simulink model "model_car"  (R2020a)
settings: Solver=VariableStepAuto  StartTime=0.0  StopTime=100  RelTol=1e-3
libraries: simulink x2
settings Model: Creator=10853  LastModifiedBy=11196

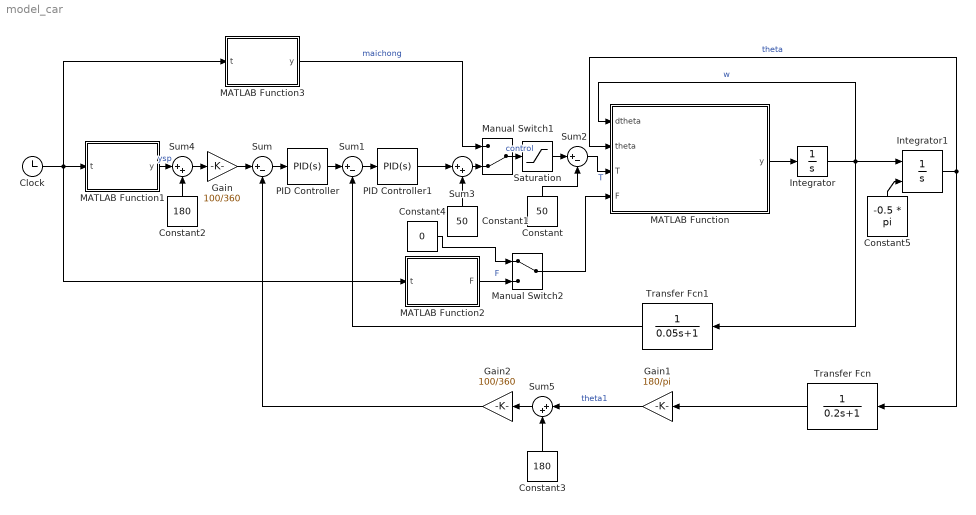
== system model_car ==
  Clock : Clock
  Constant : Constant  Value=50
  Constant1 : Constant  Value=50
  Constant2 : Constant  Value=180
  Constant3 : Constant  Value=180
  Constant4 : Constant  Value=0
  Constant5 : Constant  Value=-0.5 * pi
  Gain : Gain  Gain=100/360
  Gain1 : Gain  Gain=180/pi
  Gain2 : Gain  Gain=100/360
  Integrator : Integrator
  Integrator1 : Integrator  InitialConditionSource=external  InitialCondition=-0.5 * pi  LimitOutput=on  UpperSaturationLimit=pi  LowerSaturationLimit=-pi
  MATLAB Function : MATLAB Function  TreatAsAtomicUnit=on
  MATLAB Function1 : MATLAB Function  TreatAsAtomicUnit=on
  MATLAB Function2 : MATLAB Function  TreatAsAtomicUnit=on
  MATLAB Function3 : MATLAB Function  TreatAsAtomicUnit=on
  Manual Switch1 : ManualSwitch  CurrentSetting=0
  Manual Switch2 : ManualSwitch
  PID Controller : simulink/Continuous/PID Controller  Controller=PID  Form=Parallel  TimeDomain=Continuous-time  UseExternalTs=off  SampleTime=-1  IntegratorMethod=Forward Euler  FilterMethod=Forward Euler  ControllerParametersSource=internal  P=0.8  I=1  D=0.07  UseFilter=on  N=100  TunerSelectOption=Transfer Function Based (PID Tuner App)  InitialConditionSource=internal  InitialConditionForIntegrator=0  InitialConditionForFilter=0  DifferentiatorICPrevScaledInput=0  ExternalReset=none  TrackingMode=off  Kt=1  LimitOutput=off  UpperSaturationLimit=inf  LowerSaturationLimit=-inf  LinearizeAsGain=on  AntiWindupMode=none  Kb=1  POutMin=[]  POutMax=[]  IOutMin=[]  IOutMax=[]  DOutMin=[]  DOutMax=[]  NOutMin=[]  NOutMax=[]  SumOutMin=[]  SumOutMax=[]  SaturationOutMin=[]  SaturationOutMax=[]  PParamMin=[]  PParamMax=[]  IParamMin=[]  IParamMax=[]  DParamMin=[]  DParamMax=[]  NParamMin=[]  NParamMax=[]  KbParamMin=[]  KbParamMax=[]  KtParamMin=[]  KtParamMax=[]  KbOutMin=[]  KbOutMax=[]  KtOutMin=[]  KtOutMax=[]  IntegratorOutMin=[]  IntegratorOutMax=[]  FilterOutMin=[]  FilterOutMax=[]  SumI1OutMin=[]  SumI1OutMax=[]  SumI2OutMin=[]  SumI2OutMax=[]  SumI3OutMin=[]  SumI3OutMax=[]  SumI4OutMin=[]  SumI4OutMax=[]  SumDOutMin=[]  SumDOutMax=[]  DifferentiatorOutMin=[]  DifferentiatorOutMax=[]  FilterDiffOutCoefMin=[]  FilterDiffOutCoefMax=[]  ReciprocalOutMin=[]  ReciprocalOutMax=[]  SumDenOutMin=[]  SumDenOutMax=[]  SumNumOutMin=[]  SumNumOutMax=[]  DivideOutMin=[]  DivideOutMax=[]  UdiffTsProdOutMin=[]  UdiffTsProdOutMax=[]  NTsProdOutMin=[]  NTsProdOutMax=[]  UintegralTsProdOutMin=[]  UintegralTsProdOutMax=[]  UngainTsProdOutMin=[]  UngainTsProdOutMax=[]  IntegratorContinuousStateAttributes=''  IntegratorStateMustResolveToSignalObject=off  IntegratorRTWStateStorageClass=Auto  FilterContinuousStateAttributes=''  FilterStateMustResolveToSignalObject=off  FilterRTWStateStorageClass=Auto  ParallelPVariant=InternalParameters  IdealPVariant=Disabled  IVariant=InternalParameters  DVariant=InternalParameters  IntegratorVariant=Continuous  SatVariant=Disabled  AWVariant=Passthrough  PCopyVariant=Disabled  TRVariant=Disabled  FdbkBlocksVariant=Forward  IdealPFdbkVariant=Disabled  SatFdbkVariant=Disabled  DerivativeFilterVariant=ContFilter  NVariant=InternalParameters  NCopyVariant=Disabled  FilterICVariant=InternalICsFilter  IntegratorICVariant=InternalICs  ExternalResetVariant=Disabled  TRSumVariant=Passthrough  SumFdbkVariant=Disabled  SumVariant=Sum_PID  TsampFilterVariant=InternalTs  TsampNgainVariant=Passthrough  TsampIntegralVariant=Passthrough
  PID Controller1 : simulink/Continuous/PID Controller  Controller=PID  Form=Parallel  TimeDomain=Continuous-time  UseExternalTs=off  SampleTime=-1  IntegratorMethod=Forward Euler  FilterMethod=Forward Euler  ControllerParametersSource=internal  P=2  I=1  D=0  UseFilter=on  N=100  TunerSelectOption=Transfer Function Based (PID Tuner App)  InitialConditionSource=internal  InitialConditionForIntegrator=0  InitialConditionForFilter=0  DifferentiatorICPrevScaledInput=0  ExternalReset=none  TrackingMode=off  Kt=1  LimitOutput=off  UpperSaturationLimit=inf  LowerSaturationLimit=-inf  LinearizeAsGain=on  AntiWindupMode=none  Kb=1  POutMin=[]  POutMax=[]  IOutMin=[]  IOutMax=[]  DOutMin=[]  DOutMax=[]  NOutMin=[]  NOutMax=[]  SumOutMin=[]  SumOutMax=[]  SaturationOutMin=[]  SaturationOutMax=[]  PParamMin=[]  PParamMax=[]  IParamMin=[]  IParamMax=[]  DParamMin=[]  DParamMax=[]  NParamMin=[]  NParamMax=[]  KbParamMin=[]  KbParamMax=[]  KtParamMin=[]  KtParamMax=[]  KbOutMin=[]  KbOutMax=[]  KtOutMin=[]  KtOutMax=[]  IntegratorOutMin=[]  IntegratorOutMax=[]  FilterOutMin=[]  FilterOutMax=[]  SumI1OutMin=[]  SumI1OutMax=[]  SumI2OutMin=[]  SumI2OutMax=[]  SumI3OutMin=[]  SumI3OutMax=[]  SumI4OutMin=[]  SumI4OutMax=[]  SumDOutMin=[]  SumDOutMax=[]  DifferentiatorOutMin=[]  DifferentiatorOutMax=[]  FilterDiffOutCoefMin=[]  FilterDiffOutCoefMax=[]  ReciprocalOutMin=[]  ReciprocalOutMax=[]  SumDenOutMin=[]  SumDenOutMax=[]  SumNumOutMin=[]  SumNumOutMax=[]  DivideOutMin=[]  DivideOutMax=[]  UdiffTsProdOutMin=[]  UdiffTsProdOutMax=[]  NTsProdOutMin=[]  NTsProdOutMax=[]  UintegralTsProdOutMin=[]  UintegralTsProdOutMax=[]  UngainTsProdOutMin=[]  UngainTsProdOutMax=[]  IntegratorContinuousStateAttributes=''  IntegratorStateMustResolveToSignalObject=off  IntegratorRTWStateStorageClass=Auto  FilterContinuousStateAttributes=''  FilterStateMustResolveToSignalObject=off  FilterRTWStateStorageClass=Auto  ParallelPVariant=InternalParameters  IdealPVariant=Disabled  IVariant=InternalParameters  DVariant=InternalParameters  IntegratorVariant=Continuous  SatVariant=Disabled  AWVariant=Passthrough  PCopyVariant=Disabled  TRVariant=Disabled  FdbkBlocksVariant=Forward  IdealPFdbkVariant=Disabled  SatFdbkVariant=Disabled  DerivativeFilterVariant=ContFilter  NVariant=InternalParameters  NCopyVariant=Disabled  FilterICVariant=InternalICsFilter  IntegratorICVariant=InternalICs  ExternalResetVariant=Disabled  TRSumVariant=Passthrough  SumFdbkVariant=Disabled  SumVariant=Sum_PID  TsampFilterVariant=InternalTs  TsampNgainVariant=Passthrough  TsampIntegralVariant=Passthrough
  Saturation : Saturate  UpperLimit=100  LowerLimit=0
  Sum : Sum  Inputs=|+-
  Sum1 : Sum  Inputs=|+-
  Sum2 : Sum  Inputs=|+-
  Sum3 : Sum  Inputs=|++
  Sum4 : Sum  Inputs=|++
  Sum5 : Sum  Inputs=|++
  Transfer Fcn : TransferFcn  Denominator=[0.2 1]
  Transfer Fcn1 : TransferFcn  Denominator=[0.05 1]
  wires:
  Sum2/1 -> MATLAB Function/3(T)  "T"
  Sum1/1 -> PID Controller1/1
  Sum/1 -> PID Controller/1
  Transfer Fcn1/1 -> Sum1/2
  MATLAB Function/1(y) -> Integrator/1
  Integrator/1 -> Transfer Fcn1/1, Integrator1/1, MATLAB Function/1(dtheta)  "w"
  Constant/1 -> Sum2/2
  PID Controller1/1 -> Sum3/1
  Sum3/1 -> Manual Switch1/2
  Constant1/1 -> Sum3/2
  MATLAB Function3/1(y) -> Manual Switch1/1  "maichong"
  MATLAB Function2/1(F) -> Manual Switch2/2  "F"
  Manual Switch2/1 -> MATLAB Function/4(F)
  Constant4/1 -> Manual Switch2/1
  Manual Switch1/1 -> Saturation/1  "control"
  Saturation/1 -> Sum2/1
  Clock/1 -> MATLAB Function1/1(t), MATLAB Function2/1(t), MATLAB Function3/1(t)
  Sum4/1 -> Gain/1
  Constant2/1 -> Sum4/2
  Sum5/1 -> Gain2/1
  Constant3/1 -> Sum5/2
  Constant5/1 -> Integrator1/2
  Transfer Fcn/1 -> Gain1/1
  Integrator1/1 -> Transfer Fcn/1, MATLAB Function/2(theta)  "theta"
  MATLAB Function1/1(y) -> Sum4/1  "ysp"
  Gain/1 -> Sum/1
  Gain1/1 -> Sum5/1  "theta1"
  Gain2/1 -> Sum/2
  PID Controller/1 -> Sum1/1

== matlab function model_car/MATLAB Function ==
  data: dtheta input; theta input; T input; y output; F input
function y = fcn(dtheta,  theta, T,  F)
m = 1;
M = 100;
l = 0.5;
g = 9.8;
k1 = 1 / 3 * m * l * l;
k2 = 0.5 * l * sin(theta) * m / (M+m); 
a1 = 0.5 * m * l * sin(theta);
a2 = 0.5 * m * l * cos(theta) * dtheta * dtheta;
a3 = 0.5 * m * g * l * cos(theta);
ddtheta = (T - a3 + k2 * (a2 + F)) / (k1 - k2 * a1);
y = ddtheta;

== matlab function model_car/MATLAB Function1 ==
  data: t input; y output
function y = ysp(t)
if 0 <= t && t < 10
    y = -90;
elseif 10 <= t && t < 40
    y = 0;
elseif 40 <= t && t < 70
    y = 40;
else
    y = 90;
end

== matlab function model_car/MATLAB Function2 ==
  data: t input; F output
function F = f(t)
if (0 <= t) && (t < 5)
    F = 0;
elseif (5 <= t) && (t < 35)
    F = 5;
elseif (35 <= t) && (t < 65)
    F = -5;
else
    F = 0;
end

== matlab function model_car/MATLAB Function3 ==
  data: t input; y output
function y = maichong(t)
if 0 <= t && t < 20
    y = 50;
elseif 20 <= t && t < 20.1
    y = 58;
else
    y = 50;
end
